simulink model "CTRL_BASECTRL_GROUND_test"  (R2024b)
settings: Solver=VariableStepAuto  StartTime=0.0  StopTime=10.0  RelTol=1e-3
libraries: CTRL_BASECTRL_GROUND x1
settings Model: Creator=blatak  LastModifiedBy=blatak

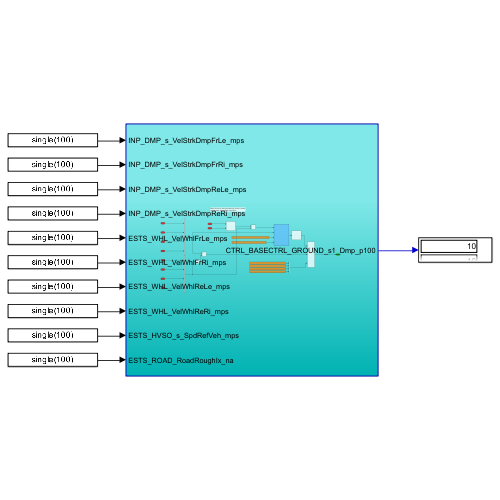
[thumbnail: Simulink's stored preview of the top-level diagram]
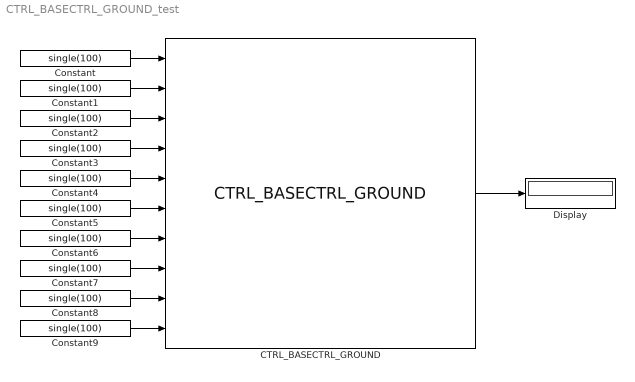
== system CTRL_BASECTRL_GROUND_test ==
  CTRL_BASECTRL_GROUND : CTRL_BASECTRL_GROUND/CTRL_BASECTRL_GROUND  SystemSampleTime=-1  VariantActivationTime=update diagram  AllowFlexibleInterface=on  Latency=0  AutoFrameSizeCalculation=off
  Constant{,1..9} (10 alike) : Constant  Value=single(100)
  Display : Display
  wires:
  Constant/1 -> CTRL_BASECTRL_GROUND/1
  Constant1/1 -> CTRL_BASECTRL_GROUND/2
  Constant2/1 -> CTRL_BASECTRL_GROUND/3
  Constant3/1 -> CTRL_BASECTRL_GROUND/4
  Constant4/1 -> CTRL_BASECTRL_GROUND/5
  Constant5/1 -> CTRL_BASECTRL_GROUND/6
  Constant6/1 -> CTRL_BASECTRL_GROUND/7
  Constant7/1 -> CTRL_BASECTRL_GROUND/8
  Constant8/1 -> CTRL_BASECTRL_GROUND/9
  Constant9/1 -> CTRL_BASECTRL_GROUND/10
  CTRL_BASECTRL_GROUND/1 -> Display/1
